simulink model "DualThresholdWindowComparator"  (R2025a)
settings: Solver=VariableStepAuto  StartTime=0.0  StopTime=10.0  RelTol=1e-3
libraries: simulink x3
settings Model: Creator=mahij  LastModifiedBy=mahij

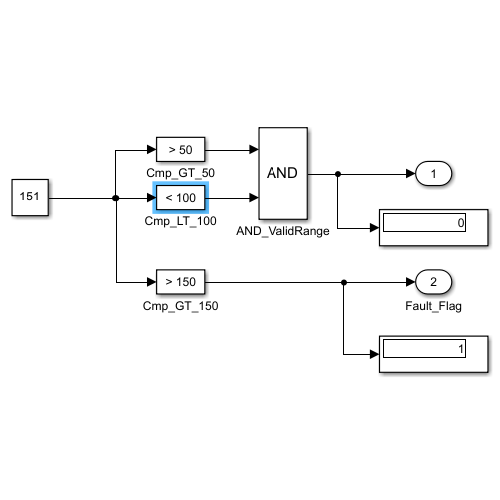
[thumbnail: Simulink's stored preview of the top-level diagram]
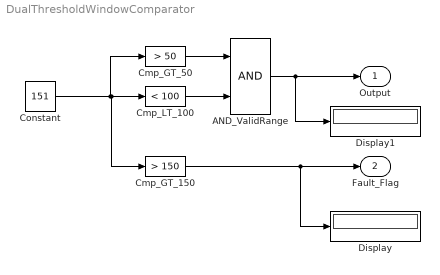
== system DualThresholdWindowComparator ==
  AND_ValidRange : Logic  AllPortsSameDT=off  OutDataTypeStr=boolean
  Cmp_GT_150 : simulink/Logic and Bit Operations/Compare To Constant  relop=>  const=150  OutDataTypeStr=boolean
  Cmp_GT_50 : simulink/Logic and Bit Operations/Compare To Constant  relop=>  const=50  OutDataTypeStr=boolean
  Cmp_LT_100 : simulink/Logic and Bit Operations/Compare To Constant  relop=<  const=100  OutDataTypeStr=boolean
  Constant : Constant  Value=151
  Display : Display
  Display1 : Display
  Output : Outport
  Fault_Flag : Outport  Port=2
  wires:
  Constant/1 -> Cmp_GT_50/1, Cmp_GT_150/1, Cmp_LT_100/1
  Cmp_GT_50/1 -> AND_ValidRange/1
  Cmp_LT_100/1 -> AND_ValidRange/2
  Cmp_GT_150/1 -> Display/1, Fault_Flag/1
  AND_ValidRange/1 -> Display1/1, Output/1
